simulink model "pade_compare"  (R2021b)
settings: Solver=VariableStepAuto  StartTime=0.0  StopTime=20000  RelTol=1e-3
undefined symbols (not defined in the file): den_P, num_P
settings Model: Creator=81702  LastModifiedBy=81702

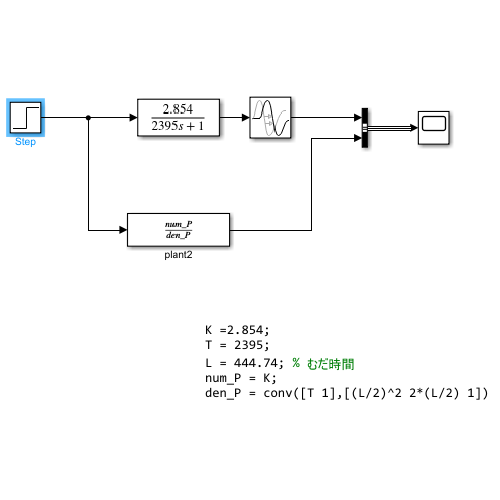
[thumbnail: Simulink's stored preview of the top-level diagram]
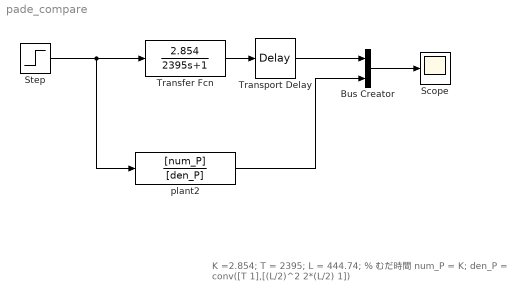
== system pade_compare ==
  note: K =2.854;
      | T = 2395;
      | L = 444.74; % むだ時間
      | num_P = K;
      | den_P = conv([T 1],[(L/2)^2 2*(L/2) 1])
  Bus Creator : BusCreator  Inputs=2
  Scope : Scope
  Step : Step  SampleTime=0
  Transfer Fcn : TransferFcn  Numerator=[2.854]  Denominator=[2395 1]
  Transport Delay : TransportDelay  DelayTime=444.74
  plant2 : TransferFcn  Numerator=[num_P]  Denominator=[den_P]
  wires:
  Bus Creator/1 -> Scope/1
  plant2/1 -> Bus Creator/2
  Transfer Fcn/1 -> Transport Delay/1
  Transport Delay/1 -> Bus Creator/1
  Step/1 -> plant2/1, Transfer Fcn/1
